simulink model "model"  (R2020b)
settings: Solver=VariableStepAuto  StartTime=0.0  StopTime=50  RelTol=1e-3
settings Model: Creator=SAGAR  LastModifiedBy=SAGAR

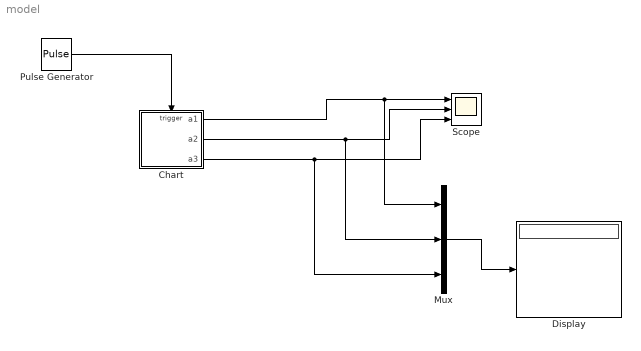
== system model ==
  Chart : Stateflow chart  TreatAsAtomicUnit=on
  Display : Display
  Mux : Mux  Inputs=3
  Pulse Generator : DiscretePulseGenerator  PulseType=Time based  Period=1  PulseWidth=50
  Scope : Scope  NumInputPorts=3
  wires:
  Pulse Generator/1 -> Chart/Trigger
  Chart/1(a1) -> Mux/1, Scope/1
  Chart/2(a2) -> Mux/2, Scope/2
  Chart/3(a3) -> Mux/3, Scope/3
  Mux/1 -> Display/1

== stateflow chart model/Chart ==
  state state1
    state ONE1
      entry:
      a1=1;
    state TWO1
      entry:
      a1=2;
    state THREE1
      entry:
      a1=3;
    state ZERO1
      entry:
      a1=0;
    state FOUR1
      entry:
      a1=4;
    ZERO1 -> ONE1 : event1
    ONE1 -> TWO1 : event1
    TWO1 -> THREE1 : event1
    THREE1 -> FOUR1 : event1
    (default) -> ZERO1
    FOUR1 -> ZERO1 : event1/{state2.event2}
  state state2
    state ONE2
      entry:
      a2=1;
    state TWO2
      entry:
      a2=2;
    state THREE2
      entry:
      a2=3;
    state ZERO2
      entry:
      a2=0;
    state FOUR2
      entry:
      a2=4;
    ZERO2 -> ONE2 : event2
    ONE2 -> TWO2 : event2
    TWO2 -> THREE2 : event2
    THREE2 -> FOUR2 : event2
    (default) -> ZERO2
    FOUR2 -> ZERO2 : event2/{state3.event3}
  state state3
    state ONE3
      entry:
      a3=1;
    state TWO3
      entry:
      a3=2;
    state THREE3
      entry:
      a3=3;
    state ZERO3
      entry:
      a3=0;
    state FOUR3
      entry:
      a3=4;
    ZERO3 -> ONE3 : event3
    ONE3 -> TWO3 : event3
    TWO3 -> THREE3 : event3
    THREE3 -> FOUR3 : event3
    (default) -> ZERO3
    FOUR3 -> ZERO3 : event3
  (default) -> state1 [order 1]
  (default) -> state2 [order 2]
  (default) -> state3 [order 3]
  data: a1 output; a2 output; a3 output
  events: event2 local FUNCTION_CALL_EVENT; event3 local FUNCTION_CALL_EVENT; event1 input RISING_EDGE_EVENT
